simulink model "Mdl_12_CloseLoop_c"  (R2018a)
settings: Solver=VariableStepAuto  StartTime=0.0  StopTime=10.0  RelTol=1e-3
undefined symbols (not defined in the file): A_mdl, B_mdl, C_mdl, D_mdl, K_mdl
settings Model: Creator=pala  LastModifiedBy=pala
settings DataIOCC: FinalStateName=xF_CL_c  SaveFinalState=on  SaveFormat=StructureWithTime  SaveState=on  SignalLogging=off  DSMLogging=off  StateSaveName=x_CL_c  TimeSaveName=t_CL_c  OutputSaveName=y_CL_c

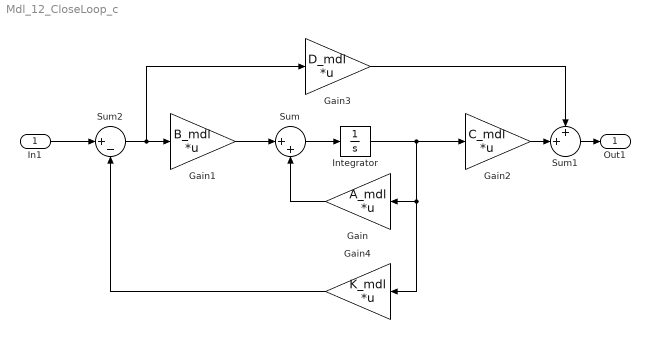
== system Mdl_12_CloseLoop_c ==
  In1 : Inport  PortDimensions=2
  Gain : Gain  Gain=A_mdl  Multiplication=Matrix(K*u)
  Gain1 : Gain  Gain=B_mdl  Multiplication=Matrix(K*u)
  Gain2 : Gain  Gain=C_mdl  Multiplication=Matrix(K*u)
  Gain3 : Gain  Gain=D_mdl  Multiplication=Matrix(K*u)
  Gain4 : Gain  Gain=K_mdl  Multiplication=Matrix(K*u)
  Integrator : Integrator
  Sum : Sum  Inputs=|++
  Sum1 : Sum  Inputs=++|
  Sum2 : Sum  Inputs=|+-
  Out1 : Outport
  wires:
  Gain/1 -> Sum/2
  Sum/1 -> Integrator/1
  Integrator/1 -> Gain2/1, Gain/1, Gain4/1
  Gain1/1 -> Sum/1
  Gain2/1 -> Sum1/2
  Sum1/1 -> Out1/1
  Gain3/1 -> Sum1/1
  In1/1 -> Sum2/1
  Sum2/1 -> Gain3/1, Gain1/1
  Gain4/1 -> Sum2/2
